simulink model "IEEE_three_phase_14Bus_test_system_with_harmonics"  (R2016a)
settings: Solver=ode15s  StartTime=0  StopTime=6/60  RelTol=1e-6
libraries: powerlib x127
(part 1 of 2)
Description:
  | 08/19/93 UW ARCHIVE           100.0  1962 W IEEE 14 Bus Test Case
  | BUS DATA FOLLOWS                            14 ITEMS
  |    1 Bus 1     HV  1  1  3 1.060    0.0      0.0      0.0    232.4   -16.9     0.0  1.060     0.0     0.0   0.0    0.0        0
  |    2 Bus 2     HV  1  1  2 1.045  -4.98     21.7     12.7     40.0    42.4     0.0  1.045    50.0   -40.0   0.0    0.0        0
  |    3 Bus 3     HV  1  1  2 1.010 -12.72     94.2     19.0      0.0    23.4     0.0  1.010    40.0     0.0   0.0    0.0        0
  |    4 Bus 4     HV  1  1  0 1.019 -10.33     47.8     -3.9      0.0     0.0     0.0  0.0       0.0     0.0   0.0    0.0        0
  |    5 Bus 5     HV  1  1  0 1.020  -8.78      7.6      1.6      0.0     0.0     0.0  0.0       0.0     0.0   0.0    0.0        0
  |    6 Bus 6     LV  1  1  2 1.070 -14.22     11.2      7.5      0.0    12.2     0.0  1.070    24.0    -6.0   0.0    0.0        0
  |    7 Bus 7     ZV  1  1  0 1.062 -13.37      0.0      0.0      0.0     0.0     0.0  0.0       0.0     0.0   0.0    0.0        0
  |    8 Bus 8     TV  1  1  2 1.090 -13.36      0.0      0.0      0.0    17.4     0.0  1.090    24.0    -6.0   0.0    0.0        0
  |    9 Bus 9     LV  1  1  0 1.056 -14.94     29.5     16.6      0.0     0.0     0.0  0.0       0.0     0.0   0.0    0.19       0
  |   10 Bus 10    LV  1  1  0 1.051 -15.10      9.0      5.8      0.0     0.0     0.0  0.0       0.0     0.0   0.0    0.0        0
  |   11 Bus 11    LV  1  1  0 1.057 -14.79      3.5      1.8      0.0     0.0     0.0  0.0       0.0     0.0   0.0    0.0        0
  |   12 Bus 12    LV  1  1  0 1.055 -15.07      6.1      1.6      0.0     0.0     0.0  0.0       0.0     0.0   0.0    0.0        0
  |   13 Bus 13    LV  1  1  0 1.050 -15.16     13.5      5.8      0.0     0.0     0.0  0.0       0.0     0.0   0.0    0.0        0
  |   14 Bus 14    LV  1  1  0 1.036 -16.04     14.9      5.0      0.0     0.0     0.0  0.0       0.0     0.0   0.0    0.0        0
  | -999
  | BRANCH DATA FOLLOWS                         20 ITEMS
  |    1    2  1  1 1 0  0.01938   0.05917     0.0528     0     0     0    0 0  0.0       0.0 0.0    0.0     0.0    0.0   0.0
  |    1    5  1  1 1 0  0.05403   0.22304     0.0492     0     0     0    0 0  0.0       0.0 0.0    0.0     0.0    0.0   0.0
  |    2    3  1  1 1 0  0.04699   0.19797     0.0438     0     0     0    0 0  0.0       0.0 0.0    0.0     0.0    0.0   0.0
  |    2    4  1  1 1 0  0.05811   0.17632     0.0340     0     0     0    0 0  0.0       0.0 0.0    0.0     0.0    0.0   0.0
  |    2    5  1  1 1 0  0.05695   0.17388     0.0346     0     0     0    0 0  0.0       0.0 0.0    0.0     0.0    0.0   0.0
  |    3    4  1  1 1 0  0.06701   0.17103     0.0128     0     0     0    0 0  0.0       0.0 0.0    0.0     0.0    0.0   0.0
  |    4    5  1  1 1 0  0.01335   0.04211     0.0        0     0     0    0 0  0.0       0.0 0.0    0.0     0.0    0.0   0.0
  |    4    7  1  1 1 0  0.0       0.20912     0.0        0     0     0    0 0  0.978     0.0 0.0    0.0     0.0    0.0   0.0
  |    4    9  1  1 1 0  0.0       0.55618     0.0        0     0     0    0 0  0.969     0.0 0.0    0.0     0.0    0.0   0.0
  |    5    6  1  1 1 0  0.0       0.25202     0.0        0     0     0    0 0  0.932     0.0 0.0    0.0     0.0    0.0   0.0
  |    6   11  1  1 1 0  0.09498   0.19890     0.0        0     0     0    0 0  0.0       0.0 0.0    0.0     0.0    0.0   0.0
  |    6   12  1  1 1 0  0.12291   0.25581     0.0        0     0     0    0 0  0.0       0.0 0.0    0.0     0.0    0.0   0.0
  |    6   13  1  1 1 0  0.06615   0.13027     0.0        0     0     0    0 0  0.0       0.0 0.0    0.0     0.0    0.0   0.0
  |    7    8  1  1 1 0  0.0       0.17615     0.0        0     0     0    0 0  0.0       0.0 0.0    0.0     0.0    0.0   0.0
  |    7    9  1  1 1 0  0.0       0.11001     0.0        0     0     0    0 0  0.0       0.0 0.0    0.0     0.0    0.0   0.0
  |    9   10  1  1 1 0  0.03181   0.08450     0.0        0     0     0    0 0  0.0       0.0 0.0    0.0     0.0    0.0   0.0
  |    9   14  1  1 1 0  0.12711   0.27038     0.0        0     0     0    0 0  0.0       0.0 0.0    0.0     0.0    0.0   0.0
  |   10   11  1  1 1 0  0.08205   0.19207     0.0        0     0     0    0 0  0.0       0.0 0.0    0.0     0.0    0.0   0.0
  |   12   13  1  1 1 0  0.22092   0.19988     0.0        0     0     0    0 0  0.0       0.0 0.0    0.0     0.0    0.0   0.0
  |   13   14  1  1 1 0  0.17093   0.34802     0.0        0     0     0    0 0  0.0       0.0 0.0    0.0     0.0    0.0   0.0
  | -999
  | LOSS ZONES FOLLOWS                     1 ITEMS
  |   1 IEEE 14 BUS
  | -99
  | INTERCHANGE DATA FOLLOWS                 1 ITEMS
  |  1    2 Bus 2     HV    0.0  999.99  IEEE14  IEEE 14 Bus Test Case
  | -9
  | TIE LINES FOLLOWS                     0 ITEMS
  | -999
  | END OF DATA
settings Model: Creator=Ramon Betancourt  LastModifiedBy=Adriana Alvarez
settings SolverCC: SolverResetMethod=Robust
settings DataIOCC: SaveFormat=Array  SignalLoggingSaveFormat=ModelDataLogs
settings DebuggingCC: SolverPrmCheckMsg=warning  FcnCallInpInsideContextMsg=UseLocalSettings
settings HardwareCC: ProdBitPerPointer=32  ProdLargestAtomicFloat=None  ProdIntDivRoundTo=Undefined  ProdEndianess=Unspecified  ProdWordSize=32  ProdHWDeviceType=32-bit Generic
settings ModelReferenceCC: PropagateSignalLabelsOutOfModel=off
settings GRTTargetCC: CombineOutputUpdateFcns=off  GRTInterface=on
settings ConfigComp: CovModelRefEnable=Off  CovSFcnEnable=off

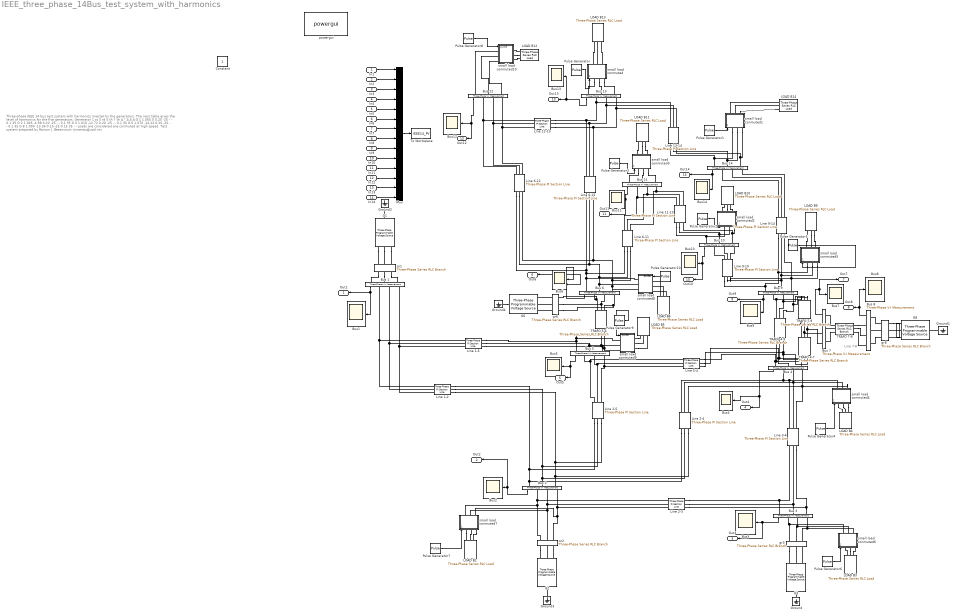
== system IEEE_three_phase_14Bus_test_system_with_harmonics ==
  note: Three-phase IEEE 14 bus test system with harmonics ijnectet by the generators. The
      | next table gives the level of harmonics for the five generators.
      |
      | Generator
      | 1 st
      | 3 rd
      | 5 th
      | 7 th
      |
      | A
      | °
      | A
      |
      | A
      |
      | A
      |
      | G 1
      | 1.060
      | 0
      | 0.20
      | -25
      | -
      | -
      | 0.1
      | 35
      |
      | G 2
      | 1.045
      | -4.98
      | 0.20
      | -25
      | -
      | -
      | 0.1
      | 35
      |
      | G 3
      | 1.010
      | -12.72
      | 0.20
      | -25
      | -
      | -
      | 0.1
      | 35
      |
      | G 6
      | 1.070
      | -14.22
      | 0.20
      | -25
      | -
      | -
      | 0.1
      | 35
      |
      | G 8
      | 1.090
      | -13.36
      | 0.10
      | -25
      | 0.15
      | 35
      | -
      | -
      |
      | Loads are considered are conmuted at high speed.
      |
      | Test system prepared by Ramon J. Betancourt rjimenez@ucol.mx
  note: Line 7-8
  In1 : Inport
  In2 : Inport  Port=2
  In3 : Inport  Port=3
  In4 : Inport  Port=4
  In5 : Inport  Port=5
  In6 : Inport  Port=6
  In7 : Inport  Port=7
  In8 : Inport  Port=8
  In9 : Inport  Port=9
  In10 : Inport  Port=10
  In11 : Inport  Port=11
  In12 : Inport  Port=12
  In13 : Inport  Port=13
  In14 : Inport  Port=14
  Bus {1..14} (14 alike) : powerlib/Measurements/Three-Phase V-I Measurement  VoltageMeasurement=phase-to-ground  SetLabelV=off  LabelV=Vabc  Vpu=on  VpuLL=off  CurrentMeasurement=no  SetLabelI=off  LabelI=Iabc  Ipu=off  Pbase=100e6  Vbase=1  OutputType=Complex  PhasorSimulation=off  PSBequivalent=0
  Bus{1..14} (14 alike) : Scope
  G1 : powerlib/Electrical Sources/Three-Phase Programmable Voltage Source  PositiveSequence="[1.06  0 60]"  VariationEntity=None  VariationType=Table of time-amplitude pairs  VariationTypeAlt=Step  VariationStep=0.5  VariationRate=10  VariationMagnitude=0.3  VariationFrequency=2  VariationTiming=[1 2]  VariationPhaseA=off  Amplitudes=[1 0.8 1.2 1.0]  TimeValues=[0 0.1 0.15 0.2]  HarmonicGeneration=on  HarmonicA=[3 0.2 -25 1]  HarmonicB=[7 0.1 35 1]  Timing="[0  6/60]"  BusType=swing  Pref=0  Qref=0  Qmin=-inf  Qmax=inf
  G2 : powerlib/Electrical Sources/Three-Phase Programmable Voltage Source  PositiveSequence="[1.045  -4.98 60]"  VariationEntity=None  VariationType=Table of time-amplitude pairs  VariationTypeAlt=Step  VariationStep=0.5  VariationRate=10  VariationMagnitude=0.3  VariationFrequency=2  VariationTiming=[1 2]  VariationPhaseA=off  Amplitudes=[1 0.8 1.2 1.0]  TimeValues=[0 0.1 0.15 0.2]  HarmonicGeneration=on  HarmonicA=[3 0.2 -25 1]  HarmonicB=[7 0.1 35 1]  Timing="[0  6/60]"  BusType=swing  Pref=0  Qref=0  Qmin=-inf  Qmax=inf
  G3 : powerlib/Electrical Sources/Three-Phase Programmable Voltage Source  PositiveSequence="[1.01  -12.72 60]"  VariationEntity=None  VariationType=Table of time-amplitude pairs  VariationTypeAlt=Step  VariationStep=0.5  VariationRate=10  VariationMagnitude=0.3  VariationFrequency=2  VariationTiming=[1 2]  VariationPhaseA=off  Amplitudes=[1 0.8 1.2 1.0]  TimeValues=[0 0.1 0.15 0.2]  HarmonicGeneration=on  HarmonicA=[3 0.2 -25 1]  HarmonicB=[7 0.1 35 1]  Timing="[0  6/60]"  BusType=swing  Pref=0  Qref=0  Qmin=-inf  Qmax=inf
  G6 : powerlib/Electrical Sources/Three-Phase Programmable Voltage Source  PositiveSequence="[1.07  -14.22 60]"  VariationEntity=None  VariationType=Table of time-amplitude pairs  VariationTypeAlt=Step  VariationStep=0.5  VariationRate=10  VariationMagnitude=0.3  VariationFrequency=2  VariationTiming=[1 2]  VariationPhaseA=off  Amplitudes=[1 0.8 1.2 1.0]  TimeValues=[0 0.1 0.15 0.2]  HarmonicGeneration=on  HarmonicA=[3 0.2 -25 1]  HarmonicB=[7 0.1 35 1]  Timing="[0  6/60]"  BusType=swing  Pref=0  Qref=0  Qmin=-inf  Qmax=inf
  G8 : powerlib/Electrical Sources/Three-Phase Programmable Voltage Source  PositiveSequence="[1.09  -13.36 60]"  VariationEntity=None  VariationType=Table of time-amplitude pairs  VariationTypeAlt=Step  VariationStep=0.5  VariationRate=10  VariationMagnitude=0.3  VariationFrequency=2  VariationTiming=[1 2]  VariationPhaseA=off  Amplitudes=[1 0.8 1.2 1.0]  TimeValues=[0 0.1 0.15 0.2]  HarmonicGeneration=on  HarmonicA=[5 0.1 -25 1]  HarmonicB=[7 0.15 35 1]  Timing="[0  20/60]"  BusType=swing  Pref=0  Qref=0  Qmin=-inf  Qmax=inf
  Ground{,1..4} (5 alike) : powerlib/Elements/Ground  LConnTagsString=a
  LOAD B10 : powerlib/Elements/Three-Phase Series RLC Load  LConnTagsString=A|B|C  Configuration=Y (grounded)  NominalVoltage=1  Vabc=[1e3 1e3 1e3]  Vabcp=[1e3 1e3 1e3]  NominalFrequency=60  UnbalancedPower=off  ActivePower=0.09  InductivePower=0.058  CapacitivePower=0  Pabc=[10e3 9e3 11e3]  QLabc=[100 90 110]  QCabc=[100 90 110]  Pabcp=[10e3 9e3 11e3]  QLabcp=[100 90 110]  QCabcp=[100 90 110]  Measurements=None  LoadType=constant Z
  LOAD B11 : powerlib/Elements/Three-Phase Series RLC Load  LConnTagsString=A|B|C  Configuration=Y (grounded)  NominalVoltage=1  Vabc=[1e3 1e3 1e3]  Vabcp=[1e3 1e3 1e3]  NominalFrequency=60  UnbalancedPower=off  ActivePower=0.035  InductivePower=0.018  CapacitivePower=0  Pabc=[10e3 9e3 11e3]  QLabc=[100 90 110]  QCabc=[100 90 110]  Pabcp=[10e3 9e3 11e3]  QLabcp=[100 90 110]  QCabcp=[100 90 110]  Measurements=None  LoadType=constant Z
  LOAD B12 : powerlib/Elements/Three-Phase Series RLC Load  LConnTagsString=A|B|C  Configuration=Y (grounded)  NominalVoltage=1  Vabc=[1e3 1e3 1e3]  Vabcp=[1e3 1e3 1e3]  NominalFrequency=60  UnbalancedPower=off  ActivePower=0.061  InductivePower=0.016  CapacitivePower=0  Pabc=[10e3 9e3 11e3]  QLabc=[100 90 110]  QCabc=[100 90 110]  Pabcp=[10e3 9e3 11e3]  QLabcp=[100 90 110]  QCabcp=[100 90 110]  Measurements=None  LoadType=constant Z
  LOAD B13 : powerlib/Elements/Three-Phase Series RLC Load  LConnTagsString=A|B|C  Configuration=Y (grounded)  NominalVoltage=1  Vabc=[1e3 1e3 1e3]  Vabcp=[1e3 1e3 1e3]  NominalFrequency=60  UnbalancedPower=off  ActivePower=0.135  InductivePower=0.058  CapacitivePower=0  Pabc=[10e3 9e3 11e3]  QLabc=[100 90 110]  QCabc=[100 90 110]  Pabcp=[10e3 9e3 11e3]  QLabcp=[100 90 110]  QCabcp=[100 90 110]  Measurements=None  LoadType=constant Z
  LOAD B14 : powerlib/Elements/Three-Phase Series RLC Load  LConnTagsString=A|B|C  Configuration=Y (grounded)  NominalVoltage=1  Vabc=[1e3 1e3 1e3]  Vabcp=[1e3 1e3 1e3]  NominalFrequency=60  UnbalancedPower=off  ActivePower=0.149  InductivePower=0.05  CapacitivePower=0  Pabc=[10e3 9e3 11e3]  QLabc=[100 90 110]  QCabc=[100 90 110]  Pabcp=[10e3 9e3 11e3]  QLabcp=[100 90 110]  QCabcp=[100 90 110]  Measurements=None  LoadType=constant Z
  LOAD B2 : powerlib/Elements/Three-Phase Series RLC Load  LConnTagsString=A|B|C  Configuration=Y (grounded)  NominalVoltage=1  Vabc=[1e3 1e3 1e3]  Vabcp=[1e3 1e3 1e3]  NominalFrequency=60  UnbalancedPower=off  ActivePower=0.217  InductivePower=0.127  CapacitivePower=0  Pabc=[10e3 9e3 11e3]  QLabc=[100 90 110]  QCabc=[100 90 110]  Pabcp=[10e3 9e3 11e3]  QLabcp=[100 90 110]  QCabcp=[100 90 110]  Measurements=None  LoadType=constant Z
  LOAD B3 : powerlib/Elements/Three-Phase Series RLC Load  LConnTagsString=A|B|C  Configuration=Y (grounded)  NominalVoltage=1  Vabc=[1e3 1e3 1e3]  Vabcp=[1e3 1e3 1e3]  NominalFrequency=60  UnbalancedPower=off  ActivePower=0.942  InductivePower=0.19  CapacitivePower=0  Pabc=[10e3 9e3 11e3]  QLabc=[100 90 110]  QCabc=[100 90 110]  Pabcp=[10e3 9e3 11e3]  QLabcp=[100 90 110]  QCabcp=[100 90 110]  Measurements=None  LoadType=constant Z
  LOAD B4 : powerlib/Elements/Three-Phase Series RLC Load  LConnTagsString=A|B|C  Configuration=Y (grounded)  NominalVoltage=1  Vabc=[1e3 1e3 1e3]  Vabcp=[1e3 1e3 1e3]  NominalFrequency=60  UnbalancedPower=off  ActivePower=0.478  InductivePower=0  CapacitivePower=0.039  Pabc=[10e3 9e3 11e3]  QLabc=[100 90 110]  QCabc=[100 90 110]  Pabcp=[10e3 9e3 11e3]  QLabcp=[100 90 110]  QCabcp=[100 90 110]  Measurements=None  LoadType=constant Z
  LOAD B5 : powerlib/Elements/Three-Phase Series RLC Load  LConnTagsString=A|B|C  Configuration=Y (grounded)  NominalVoltage=1  Vabc=[1e3 1e3 1e3]  Vabcp=[1e3 1e3 1e3]  NominalFrequency=60  UnbalancedPower=off  ActivePower=0.076  InductivePower=0.016  CapacitivePower=0  Pabc=[10e3 9e3 11e3]  QLabc=[100 90 110]  QCabc=[100 90 110]  Pabcp=[10e3 9e3 11e3]  QLabcp=[100 90 110]  QCabcp=[100 90 110]  Measurements=None  LoadType=constant Z
  LOAD B6 : powerlib/Elements/Three-Phase Series RLC Load  LConnTagsString=A|B|C  Configuration=Y (grounded)  NominalVoltage=1  Vabc=[1e3 1e3 1e3]  Vabcp=[1e3 1e3 1e3]  NominalFrequency=60  UnbalancedPower=off  ActivePower=0.112  InductivePower=0.075  CapacitivePower=0  Pabc=[10e3 9e3 11e3]  QLabc=[100 90 110]  QCabc=[100 90 110]  Pabcp=[10e3 9e3 11e3]  QLabcp=[100 90 110]  QCabcp=[100 90 110]  Measurements=None  LoadType=constant Z
  LOAD B9 : powerlib/Elements/Three-Phase Series RLC Load  LConnTagsString=A|B|C  Configuration=Y (grounded)  NominalVoltage=1  Vabc=[1e3 1e3 1e3]  Vabcp=[1e3 1e3 1e3]  NominalFrequency=60  UnbalancedPower=off  ActivePower=0.295  InductivePower=0.166  CapacitivePower=0  Pabc=[10e3 9e3 11e3]  QLabc=[100 90 110]  QCabc=[100 90 110]  Pabcp=[10e3 9e3 11e3]  QLabcp=[100 90 110]  QCabcp=[100 90 110]  Measurements=None  LoadType=constant Z
  Line 1-2 : powerlib/Elements/Three-Phase PI Section Line  LConnTagsString=a|b|c  RConnTagsString=A|B|C  Frequency=60  Resistances=[ 0.01938 0.01938]  Inductances="[ 1.5695e-04  1.5695e-04]"  Capacitances=[1.4006e-04 7.751e-9]  Length=1
  Line 1-5 : powerlib/Elements/Three-Phase PI Section Line  LConnTagsString=a|b|c  RConnTagsString=A|B|C  Frequency=60  Resistances=[ 0.05403 0.05403]  Inductances=[5.9163e-04 5.9163e-04]  Capacitances=[1.3051e-04 7.751e-9]  Length=1
  Line 11-10 : powerlib/Elements/Three-Phase PI Section Line  LConnTagsString=a|b|c  RConnTagsString=A|B|C  Frequency=60  Resistances=[ 0.08205 0.08205]  Inductances="[ 5.0948e-04  5.0948e-04]"  Capacitances=[1e-9 7.751e-9]  Length=1
  "Line 12-13 " : powerlib/Elements/Three-Phase PI Section Line  LConnTagsString=a|b|c  RConnTagsString=A|B|C  Frequency=60  Resistances=[ 0.22092 0.22092]  Inductances="[ 5.3020e-04  5.3020e-04]"  Capacitances=[1e-9 7.751e-9]  Length=1
  Line 13-14 : powerlib/Elements/Three-Phase PI Section Line  LConnTagsString=a|b|c  RConnTagsString=A|B|C  Frequency=60  Resistances=[ 0.17093 0.17093]  Inductances="[ 9.2315e-04  9.2315e-04]"  Capacitances=[1e-9 7.751e-9]  Length=1
  Line 2-3 : powerlib/Elements/Three-Phase PI Section Line  LConnTagsString=a|b|c  RConnTagsString=A|B|C  Frequency=60  Resistances="[ 0.04699  0.04699]"  Inductances="[4.6770e-04  4.6770e-04]"  Capacitances=[1.1618e-04 7.751e-9]  Length=1
  Line 2-4 : powerlib/Elements/Three-Phase PI Section Line  LConnTagsString=a|b|c  RConnTagsString=A|B|C  Frequency=60  Resistances=[ 0.05811 0.05811]  Inductances="[4.6770e-04  4.6770e-04]"  Capacitances=[9.0188e-05 7.751e-9]  Length=1
  Line 2-5 : powerlib/Elements/Three-Phase PI Section Line  LConnTagsString=a|b|c  RConnTagsString=A|B|C  Frequency=60  Resistances=[ 0.05695 0.05695]  Inductances="[4.6123e-04  4.6123e-04]"  Capacitances=[9.1779e-05 7.751e-9]  Length=1
  Line 3-4 : powerlib/Elements/Three-Phase PI Section Line  LConnTagsString=a|b|c  RConnTagsString=A|B|C  Frequency=60  Resistances=[ 0.06701 0.06701]  Inductances="[ 4.5367e-04  4.5367e-04]"  Capacitances=[3.3953e-05 7.751e-9]  Length=1
  Line 5-4 : powerlib/Elements/Three-Phase PI Section Line  LConnTagsString=a|b|c  RConnTagsString=A|B|C  Frequency=60  Resistances="[ 0.01335  0.01335]"  Inductances="[ 1.1170e-04  1.1170e-04]"  Capacitances=[1e-9 7.751e-9]  Length=1
  Line 6-11 : powerlib/Elements/Three-Phase PI Section Line  LConnTagsString=a|b|c  RConnTagsString=A|B|C  Frequency=60  Resistances=[ 0.09498 0.09498]  Inductances="[ 5.2760e-04  5.2760e-04]"  Capacitances=[1e-9 7.751e-9]  Length=1
  Line 6-12 : powerlib/Elements/Three-Phase PI Section Line  LConnTagsString=a|b|c  RConnTagsString=A|B|C  Frequency=60  Resistances=[ 0.12291 0.12291]  Inductances="[ 6.7856e-04  6.7856e-04]"  Capacitances=[1e-9 7.751e-9]  Length=1
  Line 6-13 : powerlib/Elements/Three-Phase PI Section Line  LConnTagsString=a|b|c  RConnTagsString=A|B|C  Frequency=60  Resistances=[ 0.06615 0.06615]  Inductances="[  3.4555e-04  3.4555e-04]"  Capacitances=[1e-9 7.751e-9]  Length=1
  Line 9-10 : powerlib/Elements/Three-Phase PI Section Line  LConnTagsString=a|b|c  RConnTagsString=A|B|C  Frequency=60  Resistances=[ 0.03181 0.03181]  Inductances="[ 2.2414e-04  2.2414e-04]"  Capacitances=[1e-9 7.751e-9]  Length=1
  Line 9-14 : powerlib/Elements/Three-Phase PI Section Line  LConnTagsString=a|b|c  RConnTagsString=A|B|C  Frequency=60  Resistances=[ 0.1271 0.1271]  Inductances="[ 7.1721e-04  7.1721e-04]"  Capacitances=[1e-9 7.751e-9]  Length=1
  Mux : Mux  Inputs=14
  Pulse Generator{,1..10} (11 alike) : DiscretePulseGenerator  PulseType=Time based  Period=0.005*rand  PulseWidth=10
  TRAFO 4-7 : powerlib/Elements/Three-Phase Series RLC Branch  LConnTagsString=A|B|C  RConnTagsString=A|B|C  BranchType=L  Resistance=0.01938  Inductance=5.5471e-04  Capacitance=1/0.0528/(2*pi*50)  Measurements=None
  TRAFO 4-9 : powerlib/Elements/Three-Phase Series RLC Branch  LConnTagsString=A|B|C  RConnTagsString=A|B|C  BranchType=L  Resistance=0.01938  Inductance=1.4753e-3  Capacitance=1/0.0528/(2*pi*50)  Measurements=None
  TRAFO 5-6 : powerlib/Elements/Three-Phase Series RLC Branch  LConnTagsString=A|B|C  RConnTagsString=A|B|C  BranchType=L  Resistance=0.01938  Inductance=6.685e-4  Capacitance=1/0.0528/(2*pi*50)  Measurements=None
  TRAFO 7-8 : powerlib/Elements/Three-Phase Series RLC Branch  LConnTagsString=A|B|C  RConnTagsString=A|B|C  BranchType=L  Resistance=0.01938  Inductance=4.6725e-04  Capacitance=1/0.0528/(2*pi*50)  Measurements=None
  TRAFO 7-9 : powerlib/Elements/Three-Phase Series RLC Branch  LConnTagsString=A|B|C  RConnTagsString=A|B|C  BranchType=L  Resistance=0.01938  Inductance=2.9181e-04  Capacitance=1/0.0528/(2*pi*50)  Measurements=None
  To Workspace : ToWorkspace  VariableName=IEEE14_PV  SaveFormat=Timeseries  SampleTime=-1
  gr{1..3,6,8} (5 alike) : powerlib/Elements/Three-Phase Series RLC Branch  LConnTagsString=A|B|C  RConnTagsString=A|B|C  BranchType=R  Resistance=1e-6  Inductance=1e-3  Capacitance=1e-6  Measurements=None
  powergui : powerlib/powergui  Priority=1  SimulationMode=Discrete  SolverType=Tustin  SampleTime=1e-6  frequency=60  SPID=off  DisableSnubberDevices=off  DisableRonSwitches=off  DisableVfSwitches=off  SwTol=0  DisplayEquations=off  Interpol=off  ExternalGateDelay=off  methode=off  Ts=0  FunctionMessages=off  echomessages=off  HookPort=off  EnableUseOfTLC=off  x0status=blocks  frequencyindice=60  Pbase=100e6  ErrMax=1e-4  Iterations=50  UnitsV=kV  UnitsW=MW  buscounter=0  RestoreLinks=warning  ResistiveCurrentMeasurement=off  Frange=[0:2:500]  Ylog=off  Xlog=on  ShowGrid=off  save=off  variable=ZData  structure=0  ZoomFFT=off  StartTime=0.0  cycles=1  DisplayStyle=1  fundamental=60  FreqAxis=off  MaxFrequency=1000  frequencyindicesteady=1  RmsSteady=1  display=off
  small load conmuted : Subsystem
      mask Display: image('C:\Users\Ramon Betancourt\Desktop\sun1.jpg');
  small load conmuted1 : Subsystem
      mask Display: image('C:\Users\Ramon Betancourt\Desktop\sun1.jpg');
  small load conmuted10 : Subsystem
      mask Display: image('C:\Users\Ramon Betancourt\Desktop\sun1.jpg');
  small load conmuted2 : Subsystem
      mask Display: image('C:\Users\Ramon Betancourt\Desktop\sun1.jpg');
  small load conmuted3 : Subsystem
      mask Display: image('C:\Users\Ramon Betancourt\Desktop\sun1.jpg');
  small load conmuted4 : Subsystem
      mask Display: image('C:\Users\Ramon Betancourt\Desktop\sun1.jpg');
  small load conmuted5 : Subsystem
      mask Display: image('C:\Users\Ramon Betancourt\Desktop\sun1.jpg');
  small load conmuted6 : Subsystem
      mask Display: image('C:\Users\Ramon Betancourt\Desktop\sun1.jpg');
  small load conmuted7 : Subsystem
      mask Display: image('C:\Users\Ramon Betancourt\Desktop\sun1.jpg');
  small load conmuted8 : Subsystem
      mask Display: image('C:\Users\Ramon Betancourt\Desktop\sun1.jpg');
  small load conmuted9 : Subsystem
      mask Display: image('C:\Users\Ramon Betancourt\Desktop\sun1.jpg');
  Out1 : Outport
  Out2 : Outport  Port=2
  Out3 : Outport  Port=3
  Out4 : Outport  Port=4
  Out5 : Outport  Port=5
  Out6 : Outport  Port=6
  Out7 : Outport  Port=7
  Out8 : Outport  Port=8
  Out9 : Outport  Port=9
  Out10 : Outport  Port=10
  Out11 : Outport  Port=11
  Out12 : Outport  Port=12
  Out13 : Outport  Port=13
  Out14 : Outport  Port=14
  Constant : Constant  IOType=siggen
  wires:
  Bus 2/1 -> Out2/1, Bus2/1
  Bus 8/1 -> Out8/1, Bus8/1
  Bus 3/1 -> Out3/1, Bus3/1
  Bus 4/1 -> Out4/1, Bus4/1
  Bus 5/1 -> Out5/1, Bus5/1
  Bus 6/1 -> Out6/1, Bus6/1
  Bus 7/1 -> Out7/1, Bus7/1
  Bus 9/1 -> Out9/1, Bus9/1
  Bus 10/1 -> Out10/1, Bus10/1
  Bus 11/1 -> Out11/1, Bus11/1
  Bus 12/1 -> Out12/1, Bus12/1
  Bus 13/1 -> Out13/1, Bus13/1
  Bus 14/1 -> Out14/1, Bus14/1
  Bus 1/1 -> Out1/1, Bus1/1
  In1/1 -> Mux/1
  In2/1 -> Mux/2
  In3/1 -> Mux/3
  In4/1 -> Mux/4
  In5/1 -> Mux/5
  In6/1 -> Mux/6
  In7/1 -> Mux/7
  In8/1 -> Mux/8
  In9/1 -> Mux/9
  In10/1 -> Mux/10
  In11/1 -> Mux/11
  In12/1 -> Mux/12
  In13/1 -> Mux/13
  In14/1 -> Mux/14
  Mux/1 -> To Workspace/1
  Pulse Generator/1 -> small load conmuted/1(pulse)
  Pulse Generator1/1 -> small load conmuted1/1(pulse)
  Pulse Generator2/1 -> small load conmuted2/1(pulse)
  Pulse Generator3/1 -> small load conmuted3/1(pulse)
  Pulse Generator4/1 -> small load conmuted4/1(pulse)
  Pulse Generator5/1 -> small load conmuted5/1(pulse)
  Pulse Generator6/1 -> small load conmuted6/1(pulse)
  Pulse Generator7/1 -> small load conmuted7/1(pulse)
  Pulse Generator8/1 -> small load conmuted10/1(pulse)
  Pulse Generator9/1 -> small load conmuted9/1(pulse)
  Pulse Generator10/1 -> small load conmuted8/1(pulse)
  connections:
  Line 2-4/RConn1 -- Line 2-5/RConn1 -- Line 1-2/RConn1 -- Bus 2/LConn1
  Bus 3/LConn3 -- Line 3-4/RConn3 -- Line 2-3/RConn3
  Bus 3/LConn2 -- Line 2-3/RConn2 -- Line 3-4/RConn2
  Line 1-5/LConn1 -- Line 1-2/LConn1 -- Bus 1/RConn1
  Line 1-5/LConn2 -- Line 1-2/LConn2 -- Bus 1/RConn2
  Line 1-5/LConn3 -- Line 1-2/LConn3 -- Bus 1/RConn3
  Bus 2/RConn1 -- small load conmuted7/RConn1 -- gr2/LConn1 -- Line 2-3/LConn1
  Line 2-3/LConn2 -- small load conmuted7/RConn2 -- gr2/LConn2 -- Bus 2/RConn2
  Line 2-3/LConn3 -- small load conmuted7/RConn3 -- gr2/LConn3 -- Bus 2/RConn3
  gr3/LConn1 -- small load conmuted6/RConn1 -- Bus 3/RConn1
  gr3/LConn2 -- small load conmuted6/RConn2 -- Bus 3/RConn2
  gr3/LConn3 -- small load conmuted6/RConn3 -- Bus 3/RConn3
  Line 3-4/LConn1 -- Bus 4/RConn1 -- Line 2-4/LConn1 -- small load conmuted4/RConn1
  Bus 4/RConn2 -- small load conmuted4/RConn2 -- Line 3-4/LConn2 -- Line 2-4/LConn2
  Line 5-4/LConn1 -- Line 2-5/LConn1 -- Bus 5/RConn1
  Line 5-4/LConn3 -- Line 2-5/LConn3 -- Bus 5/RConn3
  Bus 5/LConn1 -- small load conmuted9/LConn1 -- TRAFO 5-6/RConn1 -- Line 1-5/RConn1
  Bus 5/LConn2 -- TRAFO 5-6/RConn2 -- small load conmuted9/LConn2 -- Line 1-5/RConn2
  Bus 5/LConn3 -- small load conmuted9/LConn3 -- TRAFO 5-6/RConn3 -- Line 1-5/RConn3
  Line 5-4/RConn1 -- TRAFO 4-9/RConn1 -- TRAFO 4-7/RConn1 -- Bus 4/LConn1
  TRAFO 4-7/RConn2 -- Bus 4/LConn2 -- Line 5-4/RConn2 -- TRAFO 4-9/RConn2
  TRAFO 4-7/RConn3 -- Line 5-4/RConn3 -- TRAFO 4-9/RConn3 -- Bus 4/LConn3
  Bus 3/LConn1 -- Line 2-3/RConn1 -- Line 3-4/RConn1
  Line 2-5/RConn3 -- Line 1-2/RConn3 -- Line 2-4/RConn3 -- Bus 2/LConn3
  Line 2-5/RConn2 -- Line 1-2/RConn2 -- Line 2-4/RConn2 -- Bus 2/LConn2
  TRAFO 5-6/LConn1 -- gr6/RConn1 -- Bus 6/RConn1
  TRAFO 5-6/LConn2 -- gr6/RConn2 -- Bus 6/RConn2
  Line 6-12/RConn1 -- Line 6-13/RConn1 -- Line 6-11/RConn1 -- Bus 6/LConn1 -- small load conmuted8/RConn1
  Line 6-12/RConn2 -- Line 6-13/RConn2 -- Line 6-11/RConn2 -- small load conmuted8/RConn2 -- Bus 6/LConn2
  Bus 6/LConn3 -- small load conmuted8/RConn3 -- Line 6-11/RConn3 -- Line 6-12/RConn3 -- Line 6-13/RConn3
  Line 6-12/LConn1 -- Bus 12/RConn1 -- "Line 12-13 "/LConn1
  Bus 12/RConn2 -- Line 6-12/LConn2 -- "Line 12-13 "/LConn2
  Bus 12/RConn3 -- Line 6-12/LConn3 -- "Line 12-13 "/LConn3
  "Line 12-13 "/RConn1 -- Line 6-13/LConn1 -- Line 13-14/LConn1 -- Bus 13/RConn1
  "Line 12-13 "/RConn2 -- Line 6-13/LConn2 -- Line 13-14/LConn2 -- Bus 13/RConn2
  "Line 12-13 "/RConn3 -- Line 6-13/LConn3 -- Line 13-14/LConn3 -- Bus 13/RConn3
  Line 6-11/LConn1 -- Line 11-10/LConn1 -- Bus 11/RConn1
  Line 6-11/LConn2 -- Line 11-10/LConn2 -- Bus 11/RConn2
  Line 6-11/LConn3 -- Line 11-10/LConn3 -- Bus 11/RConn3
  Line 11-10/RConn2 -- small load conmuted2/LConn2 -- Bus 10/LConn2
  Line 11-10/RConn1 -- small load conmuted2/LConn1 -- Bus 10/LConn1
  Line 9-14/LConn1 -- Bus 14/RConn1
  Line 9-14/LConn2 -- Bus 14/RConn2
  Line 9-14/LConn3 -- Bus 14/RConn3
  Line 9-10/RConn1 -- small load conmuted5/LConn1 -- Line 9-14/RConn1 -- Bus 9/LConn1
  Bus 9/LConn2 -- Line 9-10/RConn2 -- small load conmuted5/LConn2 -- Line 9-14/RConn2
  Bus 9/LConn3 -- small load conmuted5/LConn3 -- Line 9-10/RConn3 -- Line 9-14/RConn3
  TRAFO 7-9/LConn1 -- Bus 9/RConn1 -- TRAFO 4-9/LConn1
  TRAFO 7-9/LConn2 -- TRAFO 4-9/LConn2 -- Bus 9/RConn2
  TRAFO 7-9/LConn3 -- TRAFO 4-9/LConn3 -- Bus 9/RConn3
  Bus 14/LConn1 -- small load conmuted1/LConn1 -- Line 13-14/RConn1
  Bus 14/LConn3 -- small load conmuted1/LConn3 -- Line 13-14/RConn3
  Line 9-10/LConn1 -- Bus 10/RConn1
  Line 9-10/LConn2 -- Bus 10/RConn2
  Line 9-10/LConn3 -- Bus 10/RConn3
  Bus 10/LConn3 -- small load conmuted2/LConn3 -- Line 11-10/RConn3
  Bus 4/RConn3 -- small load conmuted4/RConn3 -- Line 3-4/LConn3 -- Line 2-4/LConn3
  TRAFO 4-7/LConn1 -- Bus 7/RConn1 -- TRAFO 7-9/RConn1
  TRAFO 4-7/LConn2 -- Bus 7/RConn2 -- TRAFO 7-9/RConn2
  TRAFO 4-7/LConn3 -- Bus 7/RConn3 -- TRAFO 7-9/RConn3
  TRAFO 7-8/RConn1 -- Bus 7/LConn1
  TRAFO 7-8/RConn2 -- Bus 7/LConn2
  TRAFO 7-8/RConn3 -- Bus 7/LConn3
  TRAFO 7-8/LConn1 -- Bus 8/RConn1
  TRAFO 7-8/LConn2 -- Bus 8/RConn2
  TRAFO 7-8/LConn3 -- Bus 8/RConn3
  Line 5-4/LConn2 -- Line 2-5/LConn2 -- Bus 5/RConn2
  Line 13-14/RConn2 -- small load conmuted1/LConn2 -- Bus 14/LConn2
  Ground/LConn1 -- G3/LConn1
  gr3/RConn1 -- G3/RConn1
  G3/RConn2 -- gr3/RConn2
  G3/RConn3 -- gr3/RConn3
  gr8/RConn1 -- G8/RConn1
  G8/RConn2 -- gr8/RConn2
  Ground1/LConn1 -- G8/LConn1
  G8/RConn3 -- gr8/RConn3
  gr8/LConn3 -- Bus 8/LConn3
  gr8/LConn2 -- Bus 8/LConn2
  gr8/LConn1 -- Bus 8/LConn1
  Ground3/LConn1 -- G2/LConn1
  G2/RConn3 -- gr2/RConn3
  G2/RConn2 -- gr2/RConn2
  gr2/RConn1 -- G2/RConn1
  G1/LConn1 -- Ground2/LConn1
  G1/RConn1 -- gr1/RConn3
  G1/RConn2 -- gr1/RConn2
  G1/RConn3 -- gr1/RConn1
  gr1/LConn1 -- Bus 1/LConn1
  gr1/LConn2 -- Bus 1/LConn2
  gr1/LConn3 -- Bus 1/LConn3
  Ground4/LConn1 -- G6/LConn1
  TRAFO 5-6/LConn3 -- gr6/RConn3 -- Bus 6/RConn3
  gr6/LConn1 -- G6/RConn1
  gr6/LConn2 -- G6/RConn2
  gr6/LConn3 -- G6/RConn3
  small load conmuted/LConn1 -- Bus 13/LConn1
  small load conmuted/LConn2 -- Bus 13/LConn2
  small load conmuted/LConn3 -- Bus 13/LConn3
  small load conmuted/RConn1 -- LOAD B13/LConn1
  small load conmuted/RConn2 -- LOAD B13/LConn2
  small load conmuted/RConn3 -- LOAD B13/LConn3
  LOAD B14/LConn1 -- small load conmuted1/RConn1
  LOAD B14/LConn2 -- small load conmuted1/RConn2
  LOAD B14/LConn3 -- small load conmuted1/RConn3
  LOAD B10/LConn2 -- small load conmuted2/RConn2
  small load conmuted2/RConn1 -- LOAD B10/LConn1
  LOAD B10/LConn3 -- small load conmuted2/RConn3
  small load conmuted3/RConn1 -- LOAD B11/LConn1
  LOAD B11/LConn2 -- small load conmuted3/RConn2
  LOAD B11/LConn3 -- small load conmuted3/RConn3
  small load conmuted3/LConn1 -- Bus 11/LConn1
  small load conmuted3/LConn2 -- Bus 11/LConn2
  small load conmuted3/LConn3 -- Bus 11/LConn3
  small load conmuted4/LConn1 -- LOAD B4/LConn1
  small load conmuted4/LConn2 -- LOAD B4/LConn2
  small load conmuted4/LConn3 -- LOAD B4/LConn3
  small load conmuted5/RConn1 -- LOAD B9/LConn1
  LOAD B9/LConn2 -- small load conmuted5/RConn2
  LOAD B9/LConn3 -- small load conmuted5/RConn3
  small load conmuted7/LConn1 -- LOAD B2/LConn1
  LOAD B2/LConn2 -- small load conmuted7/LConn2
  small load conmuted7/LConn3 -- LOAD B2/LConn3
  LOAD B3/LConn1 -- small load conmuted6/LConn1
  small load conmuted6/LConn2 -- LOAD B3/LConn2
  small load conmuted6/LConn3 -- LOAD B3/LConn3
  LOAD B12/LConn1 -- small load conmuted10/RConn1
  small load conmuted10/RConn2 -- LOAD B12/LConn2
  small load conmuted10/RConn3 -- LOAD B12/LConn3
  small load conmuted10/LConn1 -- Bus 12/LConn1
  small load conmuted10/LConn2 -- Bus 12/LConn2
  small load conmuted10/LConn3 -- Bus 12/LConn3
  small load conmuted9/RConn1 -- LOAD B5/LConn1
  small load conmuted9/RConn2 -- LOAD B5/LConn2
  small load conmuted9/RConn3 -- LOAD B5/LConn3
  LOAD B6/LConn1 -- small load conmuted8/LConn1
  LOAD B6/LConn2 -- small load conmuted8/LConn2
  LOAD B6/LConn3 -- small load conmuted8/LConn3

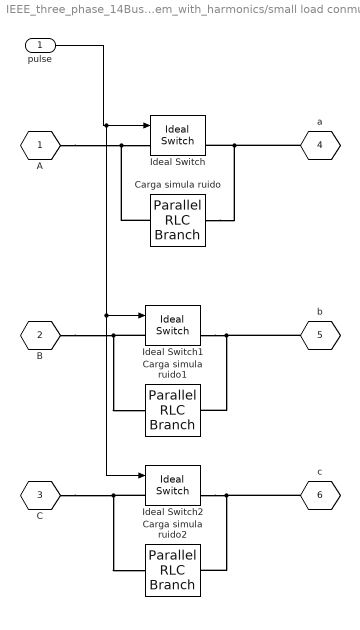
== system IEEE_three_phase_14Bus_test_system_with_harmonics/small load conmuted ==
  pulse : Inport
  Carga simula ruido : powerlib/Elements/Parallel RLC Branch  LConnTagsString=a  RConnTagsString=__new0  BranchType=RL  Resistance=2  Inductance=1e-2  SetiL0=off  InitialCurrent=0  Capacitance=0  Setx0=off  InitialVoltage=0  Measurements=None
  Carga simula ruido1 : powerlib/Elements/Parallel RLC Branch  LConnTagsString=a  RConnTagsString=__new0  BranchType=RL  Resistance=2  Inductance=1e-2  SetiL0=off  InitialCurrent=0  Capacitance=0  Setx0=off  InitialVoltage=0  Measurements=None
  Carga simula ruido2 : powerlib/Elements/Parallel RLC Branch  LConnTagsString=a  RConnTagsString=__new0  BranchType=RL  Resistance=2  Inductance=1e-2  SetiL0=off  InitialCurrent=0  Capacitance=0  Setx0=off  InitialVoltage=0  Measurements=None
  Ideal Switch : powerlib/Power Electronics/Ideal Switch  Ron=0.001  Lon=0  IC=0  Rs=1e5  Cs=inf  Measurements=on
  Ideal Switch1 : powerlib/Power Electronics/Ideal Switch  Ron=0.001  Lon=0  IC=0  Rs=1e5  Cs=inf  Measurements=on
  Ideal Switch2 : powerlib/Power Electronics/Ideal Switch  Ron=0.001  Lon=0  IC=0  Rs=1e5  Cs=inf  Measurements=on
  A : PMIOPort  Tag=PMCPort  Port=1  Side=Left
  B : PMIOPort  Tag=PMCPort  Port=2  Side=Left
  C : PMIOPort  Tag=PMCPort  Port=3  Side=Left
  a : PMIOPort  Tag=PMCPort  Port=4  Side=Right
  b : PMIOPort  Tag=PMCPort  Port=5  Side=Right
  c : PMIOPort  Tag=PMCPort  Port=6  Side=Right
  wires:
  pulse/1 -> Ideal Switch2/1, Ideal Switch1/1, Ideal Switch/1
  connections:
  A/RConn1 -- Ideal Switch/LConn1 -- Carga simula ruido/RConn1
  C/RConn1 -- Carga simula ruido2/RConn1 -- Ideal Switch2/LConn1
  B/RConn1 -- Carga simula ruido1/RConn1 -- Ideal Switch1/LConn1
  b/RConn1 -- Carga simula ruido1/LConn1 -- Ideal Switch1/RConn1
  c/RConn1 -- Carga simula ruido2/LConn1 -- Ideal Switch2/RConn1
  a/RConn1 -- Ideal Switch/RConn1 -- Carga simula ruido/LConn1

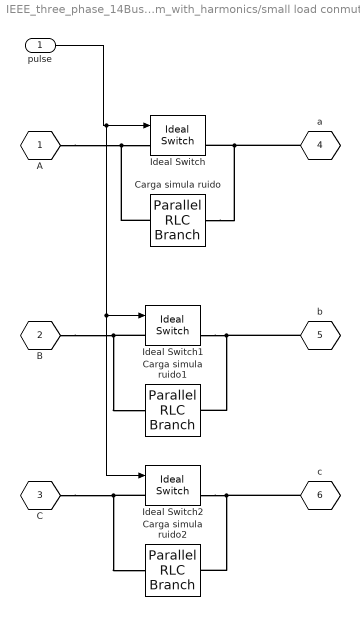
== system IEEE_three_phase_14Bus_test_system_with_harmonics/small load conmuted1 ==
  pulse : Inport
  Carga simula ruido : powerlib/Elements/Parallel RLC Branch  LConnTagsString=a  RConnTagsString=__new0  BranchType=RL  Resistance=2  Inductance=1e-2  SetiL0=off  InitialCurrent=0  Capacitance=0  Setx0=off  InitialVoltage=0  Measurements=None
  Carga simula ruido1 : powerlib/Elements/Parallel RLC Branch  LConnTagsString=a  RConnTagsString=__new0  BranchType=RL  Resistance=2  Inductance=1e-2  SetiL0=off  InitialCurrent=0  Capacitance=0  Setx0=off  InitialVoltage=0  Measurements=None
  Carga simula ruido2 : powerlib/Elements/Parallel RLC Branch  LConnTagsString=a  RConnTagsString=__new0  BranchType=RL  Resistance=2  Inductance=1e-2  SetiL0=off  InitialCurrent=0  Capacitance=0  Setx0=off  InitialVoltage=0  Measurements=None
  Ideal Switch : powerlib/Power Electronics/Ideal Switch  Ron=0.001  Lon=0  IC=0  Rs=1e5  Cs=inf  Measurements=on
  Ideal Switch1 : powerlib/Power Electronics/Ideal Switch  Ron=0.001  Lon=0  IC=0  Rs=1e5  Cs=inf  Measurements=on
  Ideal Switch2 : powerlib/Power Electronics/Ideal Switch  Ron=0.001  Lon=0  IC=0  Rs=1e5  Cs=inf  Measurements=on
  A : PMIOPort  Tag=PMCPort  Port=1  Side=Left
  B : PMIOPort  Tag=PMCPort  Port=2  Side=Left
  C : PMIOPort  Tag=PMCPort  Port=3  Side=Left
  a : PMIOPort  Tag=PMCPort  Port=4  Side=Right
  b : PMIOPort  Tag=PMCPort  Port=5  Side=Right
  c : PMIOPort  Tag=PMCPort  Port=6  Side=Right
  wires:
  pulse/1 -> Ideal Switch2/1, Ideal Switch1/1, Ideal Switch/1
  connections:
  A/RConn1 -- Ideal Switch/LConn1 -- Carga simula ruido/RConn1
  C/RConn1 -- Carga simula ruido2/RConn1 -- Ideal Switch2/LConn1
  B/RConn1 -- Carga simula ruido1/RConn1 -- Ideal Switch1/LConn1
  b/RConn1 -- Carga simula ruido1/LConn1 -- Ideal Switch1/RConn1
  c/RConn1 -- Carga simula ruido2/LConn1 -- Ideal Switch2/RConn1
  a/RConn1 -- Ideal Switch/RConn1 -- Carga simula ruido/LConn1

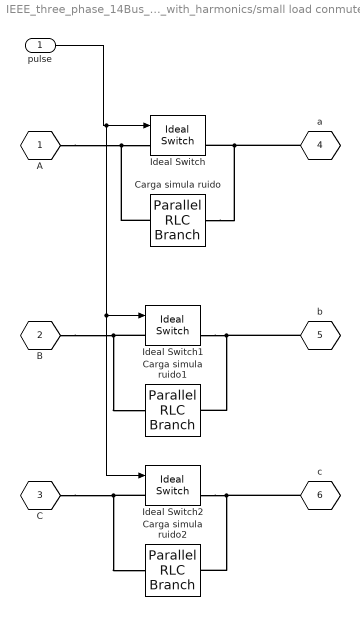
== system IEEE_three_phase_14Bus_test_system_with_harmonics/small load conmuted10 ==
  pulse : Inport
  Carga simula ruido : powerlib/Elements/Parallel RLC Branch  LConnTagsString=a  RConnTagsString=__new0  BranchType=RL  Resistance=2  Inductance=1e-2  SetiL0=off  InitialCurrent=0  Capacitance=0  Setx0=off  InitialVoltage=0  Measurements=None
  Carga simula ruido1 : powerlib/Elements/Parallel RLC Branch  LConnTagsString=a  RConnTagsString=__new0  BranchType=RL  Resistance=2  Inductance=1e-2  SetiL0=off  InitialCurrent=0  Capacitance=0  Setx0=off  InitialVoltage=0  Measurements=None
  Carga simula ruido2 : powerlib/Elements/Parallel RLC Branch  LConnTagsString=a  RConnTagsString=__new0  BranchType=RL  Resistance=2  Inductance=1e-2  SetiL0=off  InitialCurrent=0  Capacitance=0  Setx0=off  InitialVoltage=0  Measurements=None
  Ideal Switch : powerlib/Power Electronics/Ideal Switch  Ron=0.001  Lon=0  IC=0  Rs=1e5  Cs=inf  Measurements=on
  Ideal Switch1 : powerlib/Power Electronics/Ideal Switch  Ron=0.001  Lon=0  IC=0  Rs=1e5  Cs=inf  Measurements=on
  Ideal Switch2 : powerlib/Power Electronics/Ideal Switch  Ron=0.001  Lon=0  IC=0  Rs=1e5  Cs=inf  Measurements=on
  A : PMIOPort  Tag=PMCPort  Port=1  Side=Left
  B : PMIOPort  Tag=PMCPort  Port=2  Side=Left
  C : PMIOPort  Tag=PMCPort  Port=3  Side=Left
  a : PMIOPort  Tag=PMCPort  Port=4  Side=Right
  b : PMIOPort  Tag=PMCPort  Port=5  Side=Right
  c : PMIOPort  Tag=PMCPort  Port=6  Side=Right
  wires:
  pulse/1 -> Ideal Switch2/1, Ideal Switch1/1, Ideal Switch/1
  connections:
  A/RConn1 -- Ideal Switch/LConn1 -- Carga simula ruido/RConn1
  C/RConn1 -- Carga simula ruido2/RConn1 -- Ideal Switch2/LConn1
  B/RConn1 -- Carga simula ruido1/RConn1 -- Ideal Switch1/LConn1
  b/RConn1 -- Carga simula ruido1/LConn1 -- Ideal Switch1/RConn1
  c/RConn1 -- Carga simula ruido2/LConn1 -- Ideal Switch2/RConn1
  a/RConn1 -- Ideal Switch/RConn1 -- Carga simula ruido/LConn1

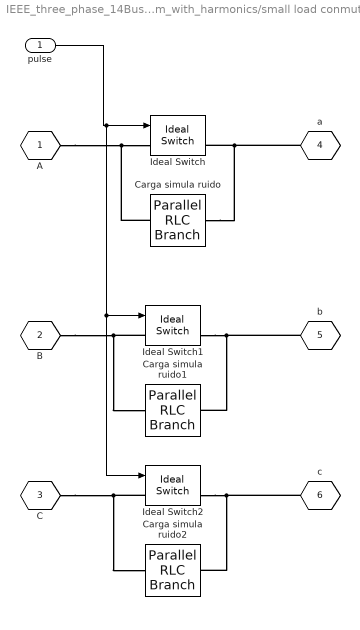
== system IEEE_three_phase_14Bus_test_system_with_harmonics/small load conmuted2 ==
  pulse : Inport
  Carga simula ruido : powerlib/Elements/Parallel RLC Branch  LConnTagsString=a  RConnTagsString=__new0  BranchType=RL  Resistance=2  Inductance=1e-2  SetiL0=off  InitialCurrent=0  Capacitance=0  Setx0=off  InitialVoltage=0  Measurements=None
  Carga simula ruido1 : powerlib/Elements/Parallel RLC Branch  LConnTagsString=a  RConnTagsString=__new0  BranchType=RL  Resistance=2  Inductance=1e-2  SetiL0=off  InitialCurrent=0  Capacitance=0  Setx0=off  InitialVoltage=0  Measurements=None
  Carga simula ruido2 : powerlib/Elements/Parallel RLC Branch  LConnTagsString=a  RConnTagsString=__new0  BranchType=RL  Resistance=2  Inductance=1e-2  SetiL0=off  InitialCurrent=0  Capacitance=0  Setx0=off  InitialVoltage=0  Measurements=None
  Ideal Switch : powerlib/Power Electronics/Ideal Switch  Ron=0.001  Lon=0  IC=0  Rs=1e5  Cs=inf  Measurements=on
  Ideal Switch1 : powerlib/Power Electronics/Ideal Switch  Ron=0.001  Lon=0  IC=0  Rs=1e5  Cs=inf  Measurements=on
  Ideal Switch2 : powerlib/Power Electronics/Ideal Switch  Ron=0.001  Lon=0  IC=0  Rs=1e5  Cs=inf  Measurements=on
  A : PMIOPort  Tag=PMCPort  Port=1  Side=Left
  B : PMIOPort  Tag=PMCPort  Port=2  Side=Left
  C : PMIOPort  Tag=PMCPort  Port=3  Side=Left
  a : PMIOPort  Tag=PMCPort  Port=4  Side=Right
  b : PMIOPort  Tag=PMCPort  Port=5  Side=Right
  c : PMIOPort  Tag=PMCPort  Port=6  Side=Right
  wires:
  pulse/1 -> Ideal Switch2/1, Ideal Switch1/1, Ideal Switch/1
  connections:
  A/RConn1 -- Ideal Switch/LConn1 -- Carga simula ruido/RConn1
  C/RConn1 -- Carga simula ruido2/RConn1 -- Ideal Switch2/LConn1
  B/RConn1 -- Carga simula ruido1/RConn1 -- Ideal Switch1/LConn1
  b/RConn1 -- Carga simula ruido1/LConn1 -- Ideal Switch1/RConn1
  c/RConn1 -- Carga simula ruido2/LConn1 -- Ideal Switch2/RConn1
  a/RConn1 -- Ideal Switch/RConn1 -- Carga simula ruido/LConn1

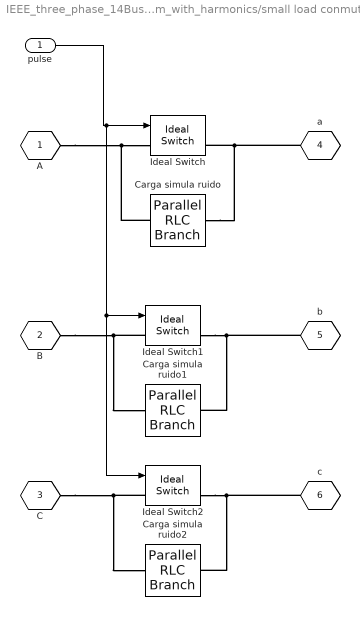
== system IEEE_three_phase_14Bus_test_system_with_harmonics/small load conmuted3 ==
  pulse : Inport
  Carga simula ruido : powerlib/Elements/Parallel RLC Branch  LConnTagsString=a  RConnTagsString=__new0  BranchType=RL  Resistance=2  Inductance=1e-2  SetiL0=off  InitialCurrent=0  Capacitance=0  Setx0=off  InitialVoltage=0  Measurements=None
  Carga simula ruido1 : powerlib/Elements/Parallel RLC Branch  LConnTagsString=a  RConnTagsString=__new0  BranchType=RL  Resistance=2  Inductance=1e-2  SetiL0=off  InitialCurrent=0  Capacitance=0  Setx0=off  InitialVoltage=0  Measurements=None
  Carga simula ruido2 : powerlib/Elements/Parallel RLC Branch  LConnTagsString=a  RConnTagsString=__new0  BranchType=RL  Resistance=2  Inductance=1e-2  SetiL0=off  InitialCurrent=0  Capacitance=0  Setx0=off  InitialVoltage=0  Measurements=None
  Ideal Switch : powerlib/Power Electronics/Ideal Switch  Ron=0.001  Lon=0  IC=0  Rs=1e5  Cs=inf  Measurements=on
  Ideal Switch1 : powerlib/Power Electronics/Ideal Switch  Ron=0.001  Lon=0  IC=0  Rs=1e5  Cs=inf  Measurements=on
  Ideal Switch2 : powerlib/Power Electronics/Ideal Switch  Ron=0.001  Lon=0  IC=0  Rs=1e5  Cs=inf  Measurements=on
  A : PMIOPort  Tag=PMCPort  Port=1  Side=Left
  B : PMIOPort  Tag=PMCPort  Port=2  Side=Left
  C : PMIOPort  Tag=PMCPort  Port=3  Side=Left
  a : PMIOPort  Tag=PMCPort  Port=4  Side=Right
  b : PMIOPort  Tag=PMCPort  Port=5  Side=Right
  c : PMIOPort  Tag=PMCPort  Port=6  Side=Right
  wires:
  pulse/1 -> Ideal Switch2/1, Ideal Switch1/1, Ideal Switch/1
  connections:
  A/RConn1 -- Ideal Switch/LConn1 -- Carga simula ruido/RConn1
  C/RConn1 -- Carga simula ruido2/RConn1 -- Ideal Switch2/LConn1
  B/RConn1 -- Carga simula ruido1/RConn1 -- Ideal Switch1/LConn1
  b/RConn1 -- Carga simula ruido1/LConn1 -- Ideal Switch1/RConn1
  c/RConn1 -- Carga simula ruido2/LConn1 -- Ideal Switch2/RConn1
  a/RConn1 -- Ideal Switch/RConn1 -- Carga simula ruido/LConn1

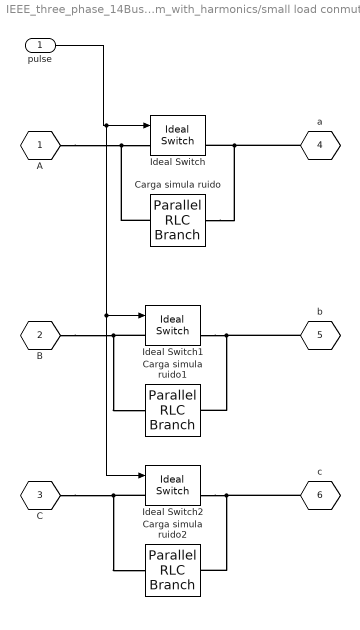
== system IEEE_three_phase_14Bus_test_system_with_harmonics/small load conmuted4 ==
  pulse : Inport
  Carga simula ruido : powerlib/Elements/Parallel RLC Branch  LConnTagsString=a  RConnTagsString=__new0  BranchType=RL  Resistance=2  Inductance=1e-2  SetiL0=off  InitialCurrent=0  Capacitance=0  Setx0=off  InitialVoltage=0  Measurements=None
  Carga simula ruido1 : powerlib/Elements/Parallel RLC Branch  LConnTagsString=a  RConnTagsString=__new0  BranchType=RL  Resistance=2  Inductance=1e-2  SetiL0=off  InitialCurrent=0  Capacitance=0  Setx0=off  InitialVoltage=0  Measurements=None
  Carga simula ruido2 : powerlib/Elements/Parallel RLC Branch  LConnTagsString=a  RConnTagsString=__new0  BranchType=RL  Resistance=2  Inductance=1e-2  SetiL0=off  InitialCurrent=0  Capacitance=0  Setx0=off  InitialVoltage=0  Measurements=None
  Ideal Switch : powerlib/Power Electronics/Ideal Switch  Ron=0.001  Lon=0  IC=0  Rs=1e5  Cs=inf  Measurements=on
  Ideal Switch1 : powerlib/Power Electronics/Ideal Switch  Ron=0.001  Lon=0  IC=0  Rs=1e5  Cs=inf  Measurements=on
  Ideal Switch2 : powerlib/Power Electronics/Ideal Switch  Ron=0.001  Lon=0  IC=0  Rs=1e5  Cs=inf  Measurements=on
  A : PMIOPort  Tag=PMCPort  Port=1  Side=Left
  B : PMIOPort  Tag=PMCPort  Port=2  Side=Left
  C : PMIOPort  Tag=PMCPort  Port=3  Side=Left
  a : PMIOPort  Tag=PMCPort  Port=4  Side=Right
  b : PMIOPort  Tag=PMCPort  Port=5  Side=Right
  c : PMIOPort  Tag=PMCPort  Port=6  Side=Right
  wires:
  pulse/1 -> Ideal Switch2/1, Ideal Switch1/1, Ideal Switch/1
  connections:
  A/RConn1 -- Ideal Switch/LConn1 -- Carga simula ruido/RConn1
  C/RConn1 -- Carga simula ruido2/RConn1 -- Ideal Switch2/LConn1
  B/RConn1 -- Carga simula ruido1/RConn1 -- Ideal Switch1/LConn1
  b/RConn1 -- Carga simula ruido1/LConn1 -- Ideal Switch1/RConn1
  c/RConn1 -- Carga simula ruido2/LConn1 -- Ideal Switch2/RConn1
  a/RConn1 -- Ideal Switch/RConn1 -- Carga simula ruido/LConn1

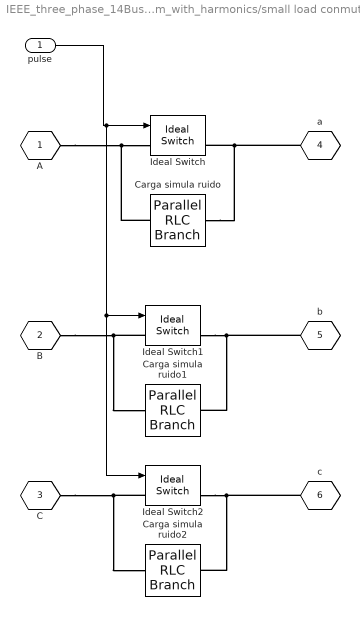
== system IEEE_three_phase_14Bus_test_system_with_harmonics/small load conmuted5 ==
  pulse : Inport
  Carga simula ruido : powerlib/Elements/Parallel RLC Branch  LConnTagsString=a  RConnTagsString=__new0  BranchType=RL  Resistance=2  Inductance=1e-2  SetiL0=off  InitialCurrent=0  Capacitance=0  Setx0=off  InitialVoltage=0  Measurements=None
  Carga simula ruido1 : powerlib/Elements/Parallel RLC Branch  LConnTagsString=a  RConnTagsString=__new0  BranchType=RL  Resistance=2  Inductance=1e-2  SetiL0=off  InitialCurrent=0  Capacitance=0  Setx0=off  InitialVoltage=0  Measurements=None
  Carga simula ruido2 : powerlib/Elements/Parallel RLC Branch  LConnTagsString=a  RConnTagsString=__new0  BranchType=RL  Resistance=2  Inductance=1e-2  SetiL0=off  InitialCurrent=0  Capacitance=0  Setx0=off  InitialVoltage=0  Measurements=None
  Ideal Switch : powerlib/Power Electronics/Ideal Switch  Ron=0.001  Lon=0  IC=0  Rs=1e5  Cs=inf  Measurements=on
  Ideal Switch1 : powerlib/Power Electronics/Ideal Switch  Ron=0.001  Lon=0  IC=0  Rs=1e5  Cs=inf  Measurements=on
  Ideal Switch2 : powerlib/Power Electronics/Ideal Switch  Ron=0.001  Lon=0  IC=0  Rs=1e5  Cs=inf  Measurements=on
  A : PMIOPort  Tag=PMCPort  Port=1  Side=Left
  B : PMIOPort  Tag=PMCPort  Port=2  Side=Left
  C : PMIOPort  Tag=PMCPort  Port=3  Side=Left
  a : PMIOPort  Tag=PMCPort  Port=4  Side=Right
  b : PMIOPort  Tag=PMCPort  Port=5  Side=Right
  c : PMIOPort  Tag=PMCPort  Port=6  Side=Right
  wires:
  pulse/1 -> Ideal Switch2/1, Ideal Switch1/1, Ideal Switch/1
  connections:
  A/RConn1 -- Ideal Switch/LConn1 -- Carga simula ruido/RConn1
  C/RConn1 -- Carga simula ruido2/RConn1 -- Ideal Switch2/LConn1
  B/RConn1 -- Carga simula ruido1/RConn1 -- Ideal Switch1/LConn1
  b/RConn1 -- Carga simula ruido1/LConn1 -- Ideal Switch1/RConn1
  c/RConn1 -- Carga simula ruido2/LConn1 -- Ideal Switch2/RConn1
  a/RConn1 -- Ideal Switch/RConn1 -- Carga simula ruido/LConn1

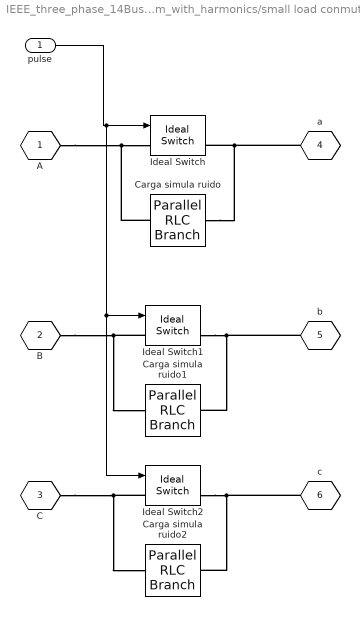
== system IEEE_three_phase_14Bus_test_system_with_harmonics/small load conmuted6 ==
  pulse : Inport
  Carga simula ruido : powerlib/Elements/Parallel RLC Branch  LConnTagsString=a  RConnTagsString=__new0  BranchType=RL  Resistance=2  Inductance=1e-2  SetiL0=off  InitialCurrent=0  Capacitance=0  Setx0=off  InitialVoltage=0  Measurements=None
  Carga simula ruido1 : powerlib/Elements/Parallel RLC Branch  LConnTagsString=a  RConnTagsString=__new0  BranchType=RL  Resistance=2  Inductance=1e-2  SetiL0=off  InitialCurrent=0  Capacitance=0  Setx0=off  InitialVoltage=0  Measurements=None
  Carga simula ruido2 : powerlib/Elements/Parallel RLC Branch  LConnTagsString=a  RConnTagsString=__new0  BranchType=RL  Resistance=2  Inductance=1e-2  SetiL0=off  InitialCurrent=0  Capacitance=0  Setx0=off  InitialVoltage=0  Measurements=None
  Ideal Switch : powerlib/Power Electronics/Ideal Switch  Ron=0.001  Lon=0  IC=0  Rs=1e5  Cs=inf  Measurements=on
  Ideal Switch1 : powerlib/Power Electronics/Ideal Switch  Ron=0.001  Lon=0  IC=0  Rs=1e5  Cs=inf  Measurements=on
  Ideal Switch2 : powerlib/Power Electronics/Ideal Switch  Ron=0.001  Lon=0  IC=0  Rs=1e5  Cs=inf  Measurements=on
  A : PMIOPort  Tag=PMCPort  Port=1  Side=Left
  B : PMIOPort  Tag=PMCPort  Port=2  Side=Left
  C : PMIOPort  Tag=PMCPort  Port=3  Side=Left
  a : PMIOPort  Tag=PMCPort  Port=4  Side=Right
  b : PMIOPort  Tag=PMCPort  Port=5  Side=Right
  c : PMIOPort  Tag=PMCPort  Port=6  Side=Right
  wires:
  pulse/1 -> Ideal Switch2/1, Ideal Switch1/1, Ideal Switch/1
  connections:
  A/RConn1 -- Ideal Switch/LConn1 -- Carga simula ruido/RConn1
  C/RConn1 -- Carga simula ruido2/RConn1 -- Ideal Switch2/LConn1
  B/RConn1 -- Carga simula ruido1/RConn1 -- Ideal Switch1/LConn1
  b/RConn1 -- Carga simula ruido1/LConn1 -- Ideal Switch1/RConn1
  c/RConn1 -- Carga simula ruido2/LConn1 -- Ideal Switch2/RConn1
  a/RConn1 -- Ideal Switch/RConn1 -- Carga simula ruido/LConn1

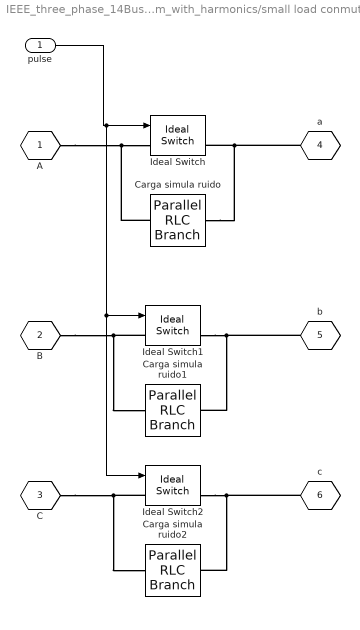
== system IEEE_three_phase_14Bus_test_system_with_harmonics/small load conmuted7 ==
  pulse : Inport
  Carga simula ruido : powerlib/Elements/Parallel RLC Branch  LConnTagsString=a  RConnTagsString=__new0  BranchType=RL  Resistance=2  Inductance=1e-2  SetiL0=off  InitialCurrent=0  Capacitance=0  Setx0=off  InitialVoltage=0  Measurements=None
  Carga simula ruido1 : powerlib/Elements/Parallel RLC Branch  LConnTagsString=a  RConnTagsString=__new0  BranchType=RL  Resistance=2  Inductance=1e-2  SetiL0=off  InitialCurrent=0  Capacitance=0  Setx0=off  InitialVoltage=0  Measurements=None
  Carga simula ruido2 : powerlib/Elements/Parallel RLC Branch  LConnTagsString=a  RConnTagsString=__new0  BranchType=RL  Resistance=2  Inductance=1e-2  SetiL0=off  InitialCurrent=0  Capacitance=0  Setx0=off  InitialVoltage=0  Measurements=None
  Ideal Switch : powerlib/Power Electronics/Ideal Switch  Ron=0.001  Lon=0  IC=0  Rs=1e5  Cs=inf  Measurements=on
  Ideal Switch1 : powerlib/Power Electronics/Ideal Switch  Ron=0.001  Lon=0  IC=0  Rs=1e5  Cs=inf  Measurements=on
  Ideal Switch2 : powerlib/Power Electronics/Ideal Switch  Ron=0.001  Lon=0  IC=0  Rs=1e5  Cs=inf  Measurements=on
  A : PMIOPort  Tag=PMCPort  Port=1  Side=Left
  B : PMIOPort  Tag=PMCPort  Port=2  Side=Left
  C : PMIOPort  Tag=PMCPort  Port=3  Side=Left
  a : PMIOPort  Tag=PMCPort  Port=4  Side=Right
  b : PMIOPort  Tag=PMCPort  Port=5  Side=Right
  c : PMIOPort  Tag=PMCPort  Port=6  Side=Right
  wires:
  pulse/1 -> Ideal Switch2/1, Ideal Switch1/1, Ideal Switch/1
  connections:
  A/RConn1 -- Ideal Switch/LConn1 -- Carga simula ruido/RConn1
  C/RConn1 -- Carga simula ruido2/RConn1 -- Ideal Switch2/LConn1
  B/RConn1 -- Carga simula ruido1/RConn1 -- Ideal Switch1/LConn1
  b/RConn1 -- Carga simula ruido1/LConn1 -- Ideal Switch1/RConn1
  c/RConn1 -- Carga simula ruido2/LConn1 -- Ideal Switch2/RConn1
  a/RConn1 -- Ideal Switch/RConn1 -- Carga simula ruido/LConn1

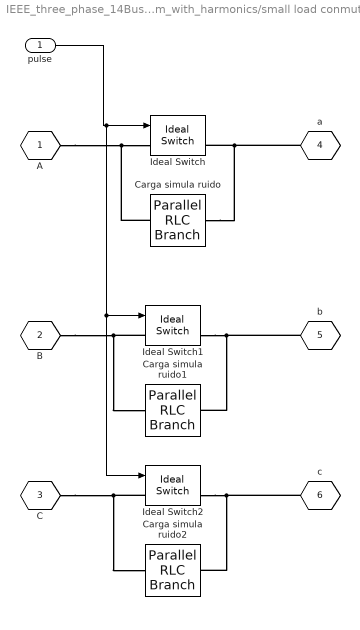
== system IEEE_three_phase_14Bus_test_system_with_harmonics/small load conmuted8 ==
  pulse : Inport
  Carga simula ruido : powerlib/Elements/Parallel RLC Branch  LConnTagsString=a  RConnTagsString=__new0  BranchType=RL  Resistance=2  Inductance=1e-2  SetiL0=off  InitialCurrent=0  Capacitance=0  Setx0=off  InitialVoltage=0  Measurements=None
  Carga simula ruido1 : powerlib/Elements/Parallel RLC Branch  LConnTagsString=a  RConnTagsString=__new0  BranchType=RL  Resistance=2  Inductance=1e-2  SetiL0=off  InitialCurrent=0  Capacitance=0  Setx0=off  InitialVoltage=0  Measurements=None
  Carga simula ruido2 : powerlib/Elements/Parallel RLC Branch  LConnTagsString=a  RConnTagsString=__new0  BranchType=RL  Resistance=2  Inductance=1e-2  SetiL0=off  InitialCurrent=0  Capacitance=0  Setx0=off  InitialVoltage=0  Measurements=None
  Ideal Switch : powerlib/Power Electronics/Ideal Switch  Ron=0.001  Lon=0  IC=0  Rs=1e5  Cs=inf  Measurements=on
  Ideal Switch1 : powerlib/Power Electronics/Ideal Switch  Ron=0.001  Lon=0  IC=0  Rs=1e5  Cs=inf  Measurements=on
  Ideal Switch2 : powerlib/Power Electronics/Ideal Switch  Ron=0.001  Lon=0  IC=0  Rs=1e5  Cs=inf  Measurements=on
  A : PMIOPort  Tag=PMCPort  Port=1  Side=Left
  B : PMIOPort  Tag=PMCPort  Port=2  Side=Left
  C : PMIOPort  Tag=PMCPort  Port=3  Side=Left
  a : PMIOPort  Tag=PMCPort  Port=4  Side=Right
  b : PMIOPort  Tag=PMCPort  Port=5  Side=Right
  c : PMIOPort  Tag=PMCPort  Port=6  Side=Right
  wires:
  pulse/1 -> Ideal Switch2/1, Ideal Switch1/1, Ideal Switch/1
  connections:
  A/RConn1 -- Ideal Switch/LConn1 -- Carga simula ruido/RConn1
  C/RConn1 -- Carga simula ruido2/RConn1 -- Ideal Switch2/LConn1
  B/RConn1 -- Carga simula ruido1/RConn1 -- Ideal Switch1/LConn1
  b/RConn1 -- Carga simula ruido1/LConn1 -- Ideal Switch1/RConn1
  c/RConn1 -- Carga simula ruido2/LConn1 -- Ideal Switch2/RConn1
  a/RConn1 -- Ideal Switch/RConn1 -- Carga simula ruido/LConn1
